simulink model "Project_Robot"  (R2018a)
settings: Solver=FixedStepAuto  StartTime=0.0  StopTime=inf  RelTol=1e-3  EnableMultiTasking=on
libraries: arduinolib x5, LCDlib x1, arduinosensorlib x1
settings Model: SimulationMode=external  ExtModeTrigDuration=2  Creator=hites  LastModifiedBy=hites
settings OptimizationCC: EnhancedBackFolding=on  PassReuseOutputArgsThreshold=0  MaxStackSize=64  OptimizeBlockOrder=speed  DifferentSizesBufferReuse=on  OptimizationCustomize=off
settings DebuggingCC: ParameterTunabilityLossMsg=error
settings HardwareCC: ProdBitPerInt=16  ProdBitPerPointer=16  ProdBitPerSizeT=16  ProdBitPerPtrDiffT=16  ProdLargestAtomicFloat=None  ProdWordSize=8  ProdHWDeviceType=Atmel->AVR  UseEmbeddedCoderFeatures=off
settings SFSimCC: MATLABDynamicMemAlloc=off
settings RTWCC: SystemTargetFile=ert.tlc  HardwareBoard=Arduino Uno  TLCOptions=-aInlineSetEventsForThisBaseRateFcn=TLC_FALSE -aSuppressMultiTaskScheduler=TLC_FALSE -aRateBasedStepFcn=1  TemplateMakefile=ert_default_tmf  GenerateReport=on  Toolchain=Arduino AVR  BuildConfiguration=Faster Runs  LaunchReport=on
settings CodeAppCC: ForceParamTrailComments=on  OperatorAnnotations=on
settings ERTTargetCC: ERTCustomFileBanners=off  SupportContinuousTime=on  SupportNonInlinedSFcns=on  RemoveResetFunc=off  SupportVariableSizeSignals=on  ModelStepFunctionPrototypeControlCompliant=off

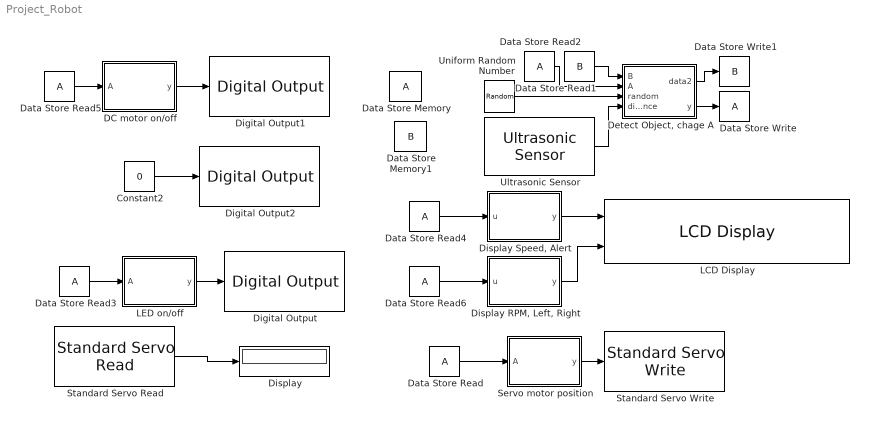
== system Project_Robot ==
  Constant2 : Constant  Value=0
  DC motor on/off : MATLAB Function  TreatAsAtomicUnit=on
  Data Store Memory : DataStoreMemory  ReadBeforeWriteMsg=warning  WriteAfterWriteMsg=warning  WriteAfterReadMsg=warning  ShowAdditionalParam=off
  Data Store Memory1 : DataStoreMemory  DataStoreName=B  ReadBeforeWriteMsg=warning  WriteAfterWriteMsg=warning  WriteAfterReadMsg=warning  ShowAdditionalParam=off
  Data Store Read{,2..6} (6 alike) : DataStoreRead
  Data Store Read1 : DataStoreRead  DataStoreName=B
  Data Store Write : DataStoreWrite
  Data Store Write1 : DataStoreWrite  DataStoreName=B
  "Detect Object, chage A" : MATLAB Function  TreatAsAtomicUnit=on
  Digital Output : arduinolib/Digital Output  pinNumber=2  blockPlatform=arduino
  Digital Output1 : arduinolib/Digital Output  pinNumber=11  blockPlatform=arduino
  Digital Output2 : arduinolib/Digital Output  pinNumber=10  blockPlatform=arduino
  Display : Display
  "Display RPM, Left, Right" : MATLAB Function  TreatAsAtomicUnit=on
  "Display Speed, Alert" : MATLAB Function  TreatAsAtomicUnit=on
  LCD Display : LCDlib/LCD Display  pins=[13, 12, 6, 5, 4, 3]
      settings: SourceProductName=LCD Library
  LED on/off : MATLAB Function  TreatAsAtomicUnit=on
  Servo motor position : MATLAB Function  TreatAsAtomicUnit=on
  Standard Servo Read : arduinolib/Standard Servo Read  pinNumber=7  sampleTime=0.5  blockPlatform=arduino
      settings: SourceProductName=Simulink Support Package for Arduino Hardware  SourceProductBaseCode=ARDUINO
  Standard Servo Write : arduinolib/Standard Servo Write  pinNumber=7  blockPlatform=arduino
      settings: SourceProductName=Simulink Support Package for Arduino Hardware
  Ultrasonic Sensor : arduinosensorlib/Ultrasonic Sensor  NumSignalPins=2  TrigPin=9  EchoPin=8  SignalPin=3  SampleTime_=0.5  blockPlatform=ARDUINO
      settings: SourceProductName=Simulink Support for Arduino Sensors
  Uniform Random Number : UniformRandomNumber  Minimum=0  SampleTime=0.5
  wires:
  Standard Servo Read/1 -> Display/1
  Ultrasonic Sensor/1 -> "Detect Object, chage A"/4(distance)
  Uniform Random Number/1 -> "Detect Object, chage A"/3(random)
  "Detect Object, chage A"/2(y) -> Data Store Write/1
  Servo motor position/1(y) -> Standard Servo Write/1
  Data Store Read/1 -> Servo motor position/1(A)
  "Detect Object, chage A"/1(data2) -> Data Store Write1/1
  Data Store Read1/1 -> "Detect Object, chage A"/1(B)
  Data Store Read2/1 -> "Detect Object, chage A"/2(A)
  LED on/off/1(y) -> Digital Output/1
  Data Store Read3/1 -> LED on/off/1(A)
  Data Store Read4/1 -> "Display Speed, Alert"/1(u)
  "Display Speed, Alert"/1(y) -> LCD Display/1
  DC motor on/off/1(y) -> Digital Output1/1
  Constant2/1 -> Digital Output2/1
  Data Store Read5/1 -> DC motor on/off/1(A)
  "Display RPM, Left, Right"/1(y) -> LCD Display/2
  Data Store Read6/1 -> "Display RPM, Left, Right"/1(u)

== matlab function Project_Robot/Servo motor position ==
  data: A input; y output
function y = fcn(A)
if A == 2
    y = 90;
else
    if A < 0.5
        y = 0;
    else
        y = 180;
    end
end

== matlab function Project_Robot/Detect Object, chage A ==
  data: B input; A input; data2 output; random input; distance input; y output
function [data2, y]= fcn( B, A, random, distance)
if  distance < 0.10
    if B == 0
        y = random;
        data2 = 1;
    else
        y = A;
        data2 = 1;
    end
else
    y = 2;
    data2 = 0;
    
end

== matlab function Project_Robot/LED on//off ==
  data: A input; y output

function y = fcn(A)
if A == 2
    y = 0;
else
    y= 1;
end

== matlab function Project_Robot/Display Speed, Alert ==
  data: u input; y output uint8
function y = fcn(u)
if u == 2
    y =uint8('DC Motor RPM');
else
    
    y = uint8('ALERT!!     ');
    
end

== matlab function Project_Robot/DC motor on//off ==
  data: A input; y output
function y = fcn(A)
if A==2
    y =1;
else
    y =0;
end

== matlab function Project_Robot/Display RPM, Left, Right ==
  data: u input; y output uint8
function y = fcn(u)
if u == 2
    y =uint8('300          ');
else
    if u< 0.5 
    y = uint8('Turning Left ');
    else
        y= uint8('Turning Right');
    end
end
